simulink model "fixpt_update_20000313_3p1"  (Simulink 4.00)
settings: Solver=FixedStepDiscrete  StartTime=0.0  StopTime=1  RelTol=1e-3
libraries: fixpt_lib_3p1 x8
settings Model: Creator=andyb  LastModifiedBy=andyb  SaveTime=off  SaveOutput=off

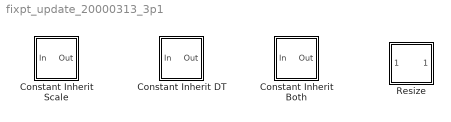
== system fixpt_update_20000313_3p1 ==
  Constant Inherit Both : Subsystem  mask(Constant with Inherited Data Type and Scaling (Obsolete)){constval=0.0, DblOver=off}
      mask prompts: constval "Constant value:"; DblOver "Override data type(s) with doubles"
      mask help: Masked Subsystem
      mask init:
      | if DblOver
      |   dboStr = 'on';
      | else
      |   dboStr = 'off';
      | end
      | set_param( [gcb, '/DTProp'], 'DblOver',dboStr);
      settings: RTWFcnNameOpts=Auto  RTWFileNameOpts=Auto
      mask Display: disp(fixpt_mask_disp_prep(constval))
  Constant Inherit DT : Subsystem  mask(Constant with Inherited Data Type (Obsolete)){constval=0.0, OutScaling=2^-1000, ConRadixGroup=Use Specified Scaling, DblOver=off}
      mask prompts: constval "Constant value:"; OutScaling "Output scaling:    Slope or [Slope Bias]    ex.  2^-9"; ConRadixGroup "Output scaling:"; DblOver "Override data type(s) with doubles"
      mask help: Masked Subsystem
      mask init:
      | if DblOver
      |   dboStr = 'on';
      | else
      |   dboStr = 'off';
      | end
      | if ConRadixGroup == 1
      |   propStr = 'Specify via dialog';
      | else
      |   propStr = 'Obtain via best precision';
      | end
      | set_param( [gcb, '/DTProp'], 'DblOver',dboStr,'PropScalingMode', propStr);
      settings: RTWFcnNameOpts=Auto  RTWFileNameOpts=Auto
      mask StyleString: edit,edit,popup(Use Specified Scaling|Best Precision: Vector-wise),checkbox
      mask Display: disp(fixpt_mask_disp_prep(constval))
  Constant Inherit Scale : Subsystem  mask(Constant with Inherited Scaling (Obsolete)){constval=0.0, OutDataType=sfix(16), DblOver=off}
      mask prompts: constval "Constant value:"; OutDataType "Output data type:     ex.  sfix(16),  uint(8),  float('single')"; DblOver "Override data type(s) with doubles"
      mask help: Masked Subsystem
      mask init:
      | if DblOver
      |   dboStr = 'on';
      | else
      |   dboStr = 'off';
      | end
      | set_param( [gcb, '/DTProp'], 'DblOver',dboStr);
      settings: RTWFcnNameOpts=Auto  RTWFileNameOpts=Auto
      mask Display: disp(fixpt_mask_disp_prep(constval))
  Resize : Subsystem  mask(Fixed-Point to Fixed-Point Resize (Obsolete)){ResizeAction=Decrease bits by half, RetainRangeOrPrecision=range, NumBits=16, RndMeth=Floor, DoSatur=off, DblOver=off, dolog=off}
      mask prompts: ResizeAction "Resize action:"; RetainRangeOrPrecision "Retain:"; NumBits "Number of Bits"; RndMeth "Round toward:"; DoSatur "Saturate to max or min when overflows occur"; DblOver "Override data type(s) with doubles"; dolog "Log minimums and maximums"
      mask help:
      | Resize the number of bits used by a Fixed-Point Blockset signal.
      |
      | This block is obsolete. Its function has been replaced by the FixPt Data Type Propagation block.  Look under the mask of this block for more information on how to use this new block to perform the same function.
      mask init:
      | ResizeAction           = get_param(gcb,'ResizeAction');
      | RetainRangeOrPrecision = get_param(gcb,'RetainRangeOrPrecision');
      | NumBits                = get_param(gcb,'NumBits');
      | RndMeth                = get_param(gcb,'RndMeth');
      | DoSatur                = get_param(gcb,'DoSatur');
      | DblOver                = get_param(gcb,'DblOver');
      | dolog                  = get_param(gcb,'dolog');
      | 
      | switch ResizeAction
      | case 'Decrease bits by half'
      |   NumBitsMult = '1/2';
      |   NumBitsAdd  = '0';
      | case 'Increase bits by twice'
      |   NumBitsMult = '2';
      |   NumBitsAdd  = '0';
      | case 'Decrease bits by specified number'
      |   NumBitsMult = '1';
      |   NumBitsAdd  = ['-(', NumBits, ')'];
      | case 'Increase bits by specified number'
      |   NumBitsMult = '1';
      |   NumBitsAdd  = NumBits;
      | case 'Set bits to specified number'
      |   NumBitsMult = '0';
      |   NumBitsAdd  = NumBits;
      | end
      | 
      | switch RetainRangeOrPrecision
      | case 'range'
      |   SlopeBase = 'PosRange1';
      | case 'precision'
      |   SlopeBase = 'Slope1';
      | end
      | 
      | set_param( [gcb, '/Conversion'], ...
      |   'RndMeth', RndMeth, ...
      |   'DoSatur', DoSatur, ...
      |   'DblOver', DblOver, ...
      |   'dolog',   dolog);
      | 
      | set_param( [gcb, '/DTProp'], ...
      |   'NumBitsMult', NumBitsMult, ...
      |   'NumBitsAdd',  NumBitsAdd, ...
      |   'SlopeBase',   SlopeBase, ...
      |   'DblOver',     DblOver);
      settings: RTWFcnNameOpts=Auto  RTWFileNameOpts=Auto
      mask Help: This block is obsolete. Its function has been replaced by the FixPt Data Type Propagation block.  Look under the mask of this block for more information on how to use this new block to perform the same function.
      mask StyleString: popup(Decrease bits by half|Decrease bits by specified number|Increase bits by twice|Increase bits by specified number|Set bits to specified number),popup(range|precision),edit,popup(Zero|Nearest|Ceiling|Floor),checkbox,checkbox,checkbox
      mask CallbackString: if any(strcmp(get_param(gcb, 'ResizeAction'), {'Decrease bits by half', 'Increase bits by twice'})), set_param(gcb, 'MaskVisibilities', {'on'; 'on'; 'off'; 'on'; 'on'; 'on'; 'on'}), else, set_param(gcb, 'MaskVisibilities', {'on'; 'on'; 'on'; 'on'; 'on'; 'on'; 'on'}), end||||||
      mask Display: fprintf('Resize')

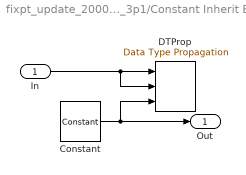
== system fixpt_update_20000313_3p1/Constant Inherit Both ==
  In : Inport  Port=1  LatchInput=off
  Constant : fixpt_lib_3p1/Sources/Constant  constval=constval  OutDataType=sfix(16)  OutScaling=2^0  ConRadixGroup=Use Specified Scaling  DblOver=off  VectInt=on
  DTProp : fixpt_lib_3p1/Data Type/Data Type Propagation  PropDataType=sfix(16)  IfRefDouble=double  IfRefSingle=single  IsSigned=IsSigned1  NumBitsBase=NumBits1  NumBitsMult=1  NumBitsAdd=0  NumBitsAllowFinal=1:128  PropScaling=2^-10  ValuesUsedBestPrec=[5 -7]  SlopeBase=Slope1  SlopeMult=1  SlopeAdd=0  BiasBase=Bias1  BiasMult=1  BiasAdd=0  DblOver=off
  Out : Outport  Port=1
  wires:
  In/1 -> DTProp/2, DTProp/1
  Constant/1 -> DTProp/3, Out/1

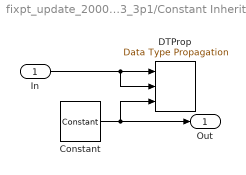
== system fixpt_update_20000313_3p1/Constant Inherit DT ==
  In : Inport  Port=1  LatchInput=off
  Constant : fixpt_lib_3p1/Sources/Constant  constval=constval  OutDataType=sfix(16)  OutScaling=2^0  ConRadixGroup=Use Specified Scaling  DblOver=off  VectInt=on
  DTProp : fixpt_lib_3p1/Data Type/Data Type Propagation  PropDataType=sfix(16)  IfRefDouble=double  IfRefSingle=single  IsSigned=IsSigned1  NumBitsBase=NumBits1  NumBitsMult=1  NumBitsAdd=0  NumBitsAllowFinal=1:128  PropScalingMode=Specify via dialog  PropScaling=OutScaling  ValuesUsedBestPrec=constval  SlopeBase=Slope1  SlopeMult=1  SlopeAdd=0  BiasBase=Bias1  BiasMult=1  BiasAdd=0  DblOver=off
  Out : Outport  Port=1
  wires:
  Constant/1 -> Out/1, DTProp/3
  In/1 -> DTProp/1, DTProp/2

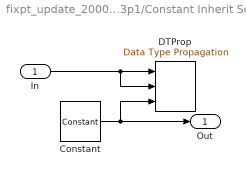
== system fixpt_update_20000313_3p1/Constant Inherit Scale ==
  In : Inport  Port=1  LatchInput=off
  Constant : fixpt_lib_3p1/Sources/Constant  constval=constval  OutDataType=sfix(16)  OutScaling=2^0  ConRadixGroup=Use Specified Scaling  DblOver=off  VectInt=on
  DTProp : fixpt_lib_3p1/Data Type/Data Type Propagation  PropDataTypeMode=Specify via dialog  PropDataType=OutDataType  IfRefDouble=double  IfRefSingle=single  IsSigned=IsSigned1  NumBitsBase=NumBits1  NumBitsMult=1  NumBitsAdd=0  NumBitsAllowFinal=1:128  PropScaling=2^-10  ValuesUsedBestPrec=[5 -7]  SlopeBase=Slope1  SlopeMult=1  SlopeAdd=0  BiasBase=Bias1  BiasMult=1  BiasAdd=0  DblOver=off
  Out : Outport  Port=1
  wires:
  In/1 -> DTProp/2, DTProp/1
  Constant/1 -> DTProp/3, Out/1

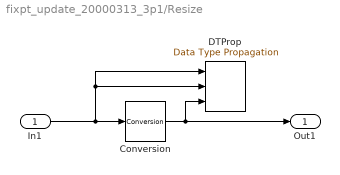
== system fixpt_update_20000313_3p1/Resize ==
  In1 : Inport  Port=1  LatchInput=off
  Conversion : fixpt_lib_3p1/Data Type/Conversion  ConvertRealWorld=Real World Value  OutDataType=sfix(16)  OutScaling=2^-10  DoSatur=off  DblOver=off  dolog=off
  DTProp : fixpt_lib_3p1/Data Type/Data Type Propagation  PropDataType=sfix(16)  IfRefDouble=double  IfRefSingle=single  IsSigned=IsSigned1  NumBitsBase=NumBits1  NumBitsMult=1/2  NumBitsAdd=0  NumBitsAllowFinal=1:128  PropScaling=2^-10  ValuesUsedBestPrec=[5 -7]  SlopeBase=PosRange1  SlopeMult=1  SlopeAdd=0  BiasBase=Bias1  BiasMult=1  BiasAdd=0  DblOver=off
  Out1 : Outport  Port=1
  wires:
  In1/1 -> Conversion/1, DTProp/1, DTProp/2
  Conversion/1 -> Out1/1, DTProp/3
